simulink model "Q7_IdealTransfo2"  (R2019b)
settings: Solver=daessc  StartTime=0.0  StopTime=10.0  RelTol=1e-3  AbsTol=1e-3  EnableMultiTasking=on
libraries: powerlib x11, powerlib_meascontrol x2
settings Model: Creator=FranciscoM  LastModifiedBy=F Gonzalez-Longatt
settings SolverCC: AutoScaleAbsTol=off
settings DataIOCC: LimitDataPoints=on  ReturnWorkspaceOutputs=off
settings OptimizationCC: LifeSpan=inf
settings DebuggingCC: AllowSymbolicDim=off  SFUnexpectedBacktrackingDiag=warning  SFNoUnconditionalDefaultTransitionDiag=warning  SFExecutionAtInitializationDiag=none  ArithmeticOperatorsInVariantConditions=warning
settings SFSimCC: SimUseLocalCustomCode=off  CustomCodeUndefinedFunction=UseInterfaceOnly
settings RTWCC: RTWUseLocalCustomCode=off
settings CodeAppCC: StateflowObjectComments=on
settings GRTTargetCC: TargetLangStandard=C89/C90 (ANSI)  GeneratePreprocessorConditionals=Disable all
settings ConfigComp: CovMetricSettings=dw  CovHtmlReporting=on  CovSaveCumulativeToWorkspaceVar=on  CovSaveSingleToWorkspaceVar=on  CovExternalEMLEnable=off  CovSFcnEnable=off
settings SimscapeCC: SimscapeNormalizeSystem=off  SimscapeLogType=all  SimscapeLogDataHistory=10000

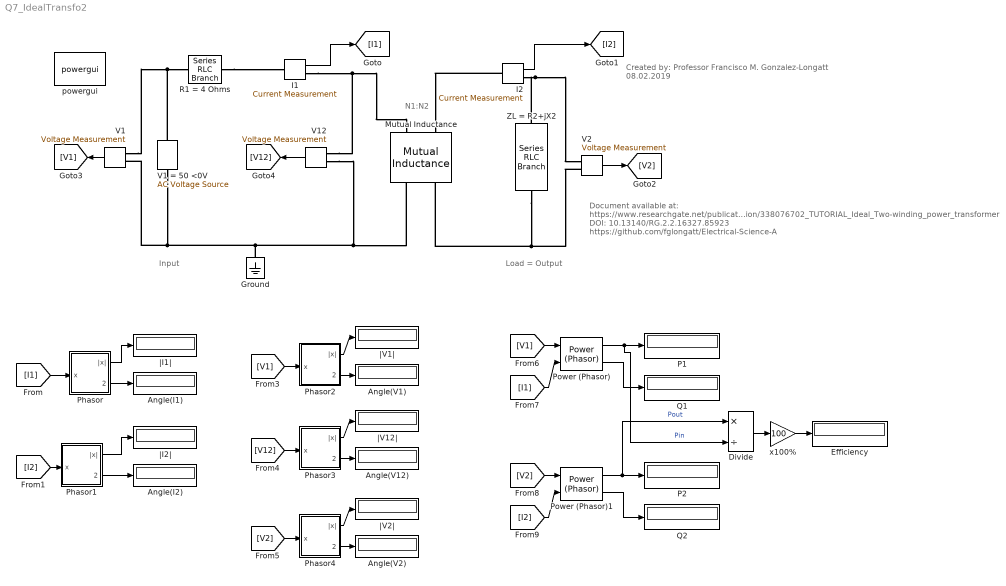
== system Q7_IdealTransfo2 ==
  note: Document available at: https://www.researchgate.net/publication/338076702_TUTORIAL_Ideal_Two-winding_power_transformer
      | DOI: 10.13140/RG.2.2.16327.85923
      | https://github.com/fglongatt/Electrical-Science-A
  note: N1:N2
  note: Load = Output
  note: Created by: Professor Francisco M. Gonzalez-Longatt
      | 08.02.2019
  note: Input
  Angle(I1) : Display
  Angle(I2) : Display
  Angle(V1) : Display
  Angle(V12) : Display
  Angle(V2) : Display
  Divide : Product  Inputs=*/
  Efficiency : Display
  Ground : powerlib/Elements/Ground  LConnTagsString=a
      settings: SourceProductName=Simscape Electrical
  I1 : powerlib/Measurements/Current Measurement  PhasorSimulation=on  OutputType=Complex  PSBequivalent=0
      settings: SourceProductName=Simscape Electrical
  I2 : powerlib/Measurements/Current Measurement  PhasorSimulation=on  OutputType=Complex  PSBequivalent=0
      settings: SourceProductName=Simscape Electrical
  Mutual Inductance : powerlib/Elements/Mutual Inductance  LConnTagsString=a|b  RConnTagsString=A|B  TypeOfMutual=Two or three windings with equal mutual terms  NumberOfWindings=3  SelfImpedance1=[0.00000001 2.0e-03]  SelfImpedance2=[ 0.0000001 5.0e-03]  ThreeWindings=off  SelfImpedance3=[ 1.1 1.1e-03]  MutualImpedance=[0.000001 3.0e-03]  InductanceMatrix="[1.0 0.9  0.9 ;  0.9 1.0  0.9;  0.9 0.9 1.0 ] * 1e-3"  ResistanceMatrix="[1.0 0.9  0.9 ;  0.9 1.0  0.9;  0.9 0.9 1.0 ]"  Measurements=None
      settings: AttributesFormatString=\n  SourceProductName=Simscape Electrical  SourceProductBaseCode=PS
  P1 : Display
  P2 : Display
  Phasor : Subsystem  TreatAsAtomicUnit=on
  Phasor1 : Subsystem  TreatAsAtomicUnit=on
  Phasor2 : Subsystem  TreatAsAtomicUnit=on
  Phasor3 : Subsystem  TreatAsAtomicUnit=on
  Phasor4 : Subsystem  TreatAsAtomicUnit=on
  Power (Phasor) : powerlib_meascontrol/Measurements/Power (Phasor)
      settings: SourceProductName=Simscape Electrical  SourceProductBaseCode=PS
  Power (Phasor)1 : powerlib_meascontrol/Measurements/Power (Phasor)
      settings: SourceProductName=Simscape Electrical  SourceProductBaseCode=PS
  Q1 : Display
  Q2 : Display
  R1 = 4 Ohms : powerlib/Elements/Series RLC Branch  LConnTagsString=__new0  RConnTagsString=__new0  BranchType=R  Resistance=4  Inductance=1e-3  SetiL0=off  InitialCurrent=0  Capacitance=inf  Setx0=off  InitialVoltage=0  Measurements=None
      settings: SourceProductName=Simscape Electrical
  V1 : powerlib/Measurements/Voltage Measurement  PhasorSimulation=on  OutputType=Complex  PSBequivalent=0
      settings: SourceProductName=Simscape Electrical
  V1 = 50 <0V : powerlib/Electrical Sources/AC Voltage Source  Amplitude=50*sqrt(2)  Phase=180  Frequency=159.1549  SampleTime=0  Measurements=None  BusType=swing  Pref=10e3  Qref=0  Qmin=-inf  Qmax=+inf
      settings: SourceProductName=Simscape Electrical
  V12 : powerlib/Measurements/Voltage Measurement  PhasorSimulation=on  OutputType=Complex  PSBequivalent=0
      settings: SourceProductName=Simscape Electrical
  V2 : powerlib/Measurements/Voltage Measurement  PhasorSimulation=on  OutputType=Complex  PSBequivalent=0
      settings: SourceProductName=Simscape Electrical
  ZL = R2+jX2 : powerlib/Elements/Series RLC Branch  LConnTagsString=__new0  RConnTagsString=__new0  BranchType=RC  Resistance=10  Inductance=1.75/(2*pi*50)  SetiL0=off  InitialCurrent=0  Capacitance=20e-6  Setx0=off  InitialVoltage=0  Measurements=None
      settings: SourceProductName=Simscape Electrical
  powergui : powerlib/powergui  Priority=1  SimulationMode=Phasor  SampleTime=50e-6  frequency=159.1549  Iterations=50  frequencyindice=159.1549  Pbase=100e6  ErrMax=1e-4  UnitsV=kV  UnitsW=MW  buscounter=0  FunctionMessages=off  echomessages=off  EnableUseOfTLC=off  CurrentSourceSwitches=off  DisableSnubberDevices=off  DisableRonSwitches=off  DisableVfSwitches=off  DisplayEquations=off  AutomaticDiscreteSolvers=off  SolverType=Tustin/Backward Euler (TBE)  Interpol=off  ExternalGateDelay=off  methode=off  Ts=100  x0status=blocks  SPID=off  SwTol=0  HookPort=off  NonlinearTolerance=1e-4  nMaxIteration=100  ContinueOnMaxIteration=off  RestoreLinks=warning  ResistiveCurrentMeasurement=off  Frange=[0:2:500]  Ylog=off  Xlog=on  ShowGrid=off  save=off  variable=ZData  structure=0  ZoomFFT=off  StartTime=0.0  cycles=1  DisplayStyle=1  fundamental=60  FreqAxis=off  MaxFrequency=1000  frequencyindicesteady=1  RmsSteady=2  display=off
      settings: SourceProductName=Simscape Electrical
  x100% : Gain  Gain=100
  |I1| : Display
  |I2| : Display
  |V12| : Display
  |V1| : Display
  |V2| : Display
  wires:
  [I1] -> Phasor/1(x)
  Power (Phasor)1/2 -> Q2/1
  Phasor1/2(angle(x)) -> Angle(I2)/1
  Power (Phasor)/2 -> Q1/1
  [V12] -> Phasor3/1(x)
  Phasor4/2(angle(x)) -> Angle(V2)/1
  Phasor1/1(|x|) -> |I2|/1
  [I1] -> Power (Phasor)/2
  Phasor2/2(angle(x)) -> Angle(V1)/1
  Phasor3/1(|x|) -> |V12|/1
  Phasor/2(angle(x)) -> Angle(I1)/1
  [I2] -> Power (Phasor)1/2
  Phasor2/1(|x|) -> |V1|/1
  [I2] -> Phasor1/1(x)
  x100%/1 -> Efficiency/1
  Divide/1 -> x100%/1
  Phasor4/1(|x|) -> |V2|/1
  [V1] -> Phasor2/1(x)
  Phasor/1(|x|) -> |I1|/1
  Power (Phasor)1/1 -> Divide/1, P2/1  "Pout"
  [V2] -> Power (Phasor)1/1
  Power (Phasor)/1 -> Divide/2, P1/1  "Pin"
  [V2] -> Phasor4/1(x)
  Phasor3/2(angle(x)) -> Angle(V12)/1
  [V1] -> Power (Phasor)/1
  V12/1 -> [V12]
  V1/1 -> [V1]
  V2/1 -> [V2]
  I2/1 -> [I2]
  I1/1 -> [I1]
  connections:
  V1/LConn1 -- V1 = 50 <0V/RConn1 -- R1 = 4 Ohms/LConn1
  V12/LConn2 -- Ground/LConn1 -- V1 = 50 <0V/LConn1 -- V1/LConn2 -- Mutual Inductance/RConn1
  V12/LConn1 -- Mutual Inductance/LConn1 -- I1/RConn1
  I2/RConn1 -- ZL = R2+jX2/LConn1 -- V2/LConn1
  V2/LConn2 -- ZL = R2+jX2/RConn1 -- Mutual Inductance/RConn2
  R1 = 4 Ohms/RConn1 -- I1/LConn1
  I2/LConn1 -- Mutual Inductance/LConn2

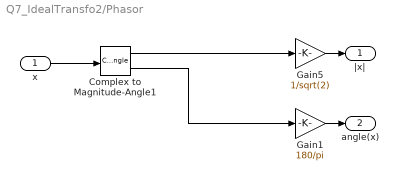
== system Q7_IdealTransfo2/Phasor ==
  x : Inport
  Complex to Magnitude-Angle1 : ComplexToMagnitudeAngle
  Gain1 : Gain  Gain=180/pi
  Gain5 : Gain  Gain=1/sqrt(2)
  |x| : Outport  VectorParamsAs1DForOutWhenUnconnected=off
  angle(x) : Outport  Port=2  VectorParamsAs1DForOutWhenUnconnected=off
  wires:
  x/1 -> Complex to Magnitude-Angle1/1
  Complex to Magnitude-Angle1/1 -> Gain5/1
  Gain5/1 -> |x|/1
  Complex to Magnitude-Angle1/2 -> Gain1/1
  Gain1/1 -> angle(x)/1

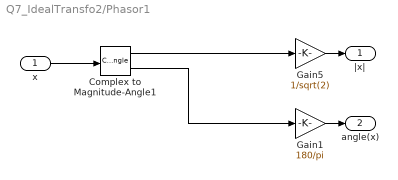
== system Q7_IdealTransfo2/Phasor1 ==
  x : Inport
  Complex to Magnitude-Angle1 : ComplexToMagnitudeAngle
  Gain1 : Gain  Gain=180/pi
  Gain5 : Gain  Gain=1/sqrt(2)
  |x| : Outport  VectorParamsAs1DForOutWhenUnconnected=off
  angle(x) : Outport  Port=2  VectorParamsAs1DForOutWhenUnconnected=off
  wires:
  x/1 -> Complex to Magnitude-Angle1/1
  Complex to Magnitude-Angle1/1 -> Gain5/1
  Gain5/1 -> |x|/1
  Complex to Magnitude-Angle1/2 -> Gain1/1
  Gain1/1 -> angle(x)/1

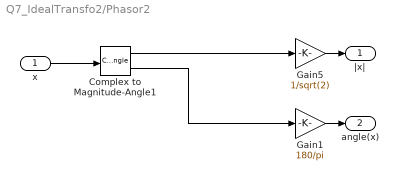
== system Q7_IdealTransfo2/Phasor2 ==
  x : Inport
  Complex to Magnitude-Angle1 : ComplexToMagnitudeAngle
  Gain1 : Gain  Gain=180/pi
  Gain5 : Gain  Gain=1/sqrt(2)
  |x| : Outport  VectorParamsAs1DForOutWhenUnconnected=off
  angle(x) : Outport  Port=2  VectorParamsAs1DForOutWhenUnconnected=off
  wires:
  x/1 -> Complex to Magnitude-Angle1/1
  Complex to Magnitude-Angle1/1 -> Gain5/1
  Gain5/1 -> |x|/1
  Complex to Magnitude-Angle1/2 -> Gain1/1
  Gain1/1 -> angle(x)/1

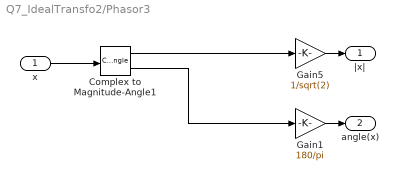
== system Q7_IdealTransfo2/Phasor3 ==
  x : Inport
  Complex to Magnitude-Angle1 : ComplexToMagnitudeAngle
  Gain1 : Gain  Gain=180/pi
  Gain5 : Gain  Gain=1/sqrt(2)
  |x| : Outport  VectorParamsAs1DForOutWhenUnconnected=off
  angle(x) : Outport  Port=2  VectorParamsAs1DForOutWhenUnconnected=off
  wires:
  x/1 -> Complex to Magnitude-Angle1/1
  Complex to Magnitude-Angle1/1 -> Gain5/1
  Gain5/1 -> |x|/1
  Complex to Magnitude-Angle1/2 -> Gain1/1
  Gain1/1 -> angle(x)/1

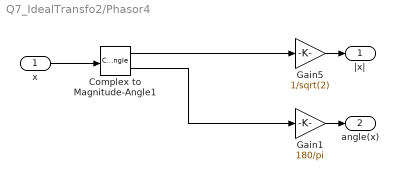
== system Q7_IdealTransfo2/Phasor4 ==
  x : Inport
  Complex to Magnitude-Angle1 : ComplexToMagnitudeAngle
  Gain1 : Gain  Gain=180/pi
  Gain5 : Gain  Gain=1/sqrt(2)
  |x| : Outport  VectorParamsAs1DForOutWhenUnconnected=off
  angle(x) : Outport  Port=2  VectorParamsAs1DForOutWhenUnconnected=off
  wires:
  x/1 -> Complex to Magnitude-Angle1/1
  Complex to Magnitude-Angle1/1 -> Gain5/1
  Gain5/1 -> |x|/1
  Complex to Magnitude-Angle1/2 -> Gain1/1
  Gain1/1 -> angle(x)/1
